simulink model "OCTModel_bandLin"  (R2020a)
settings: Solver=ode23s  StartTime=0.0  StopTime=simParams.duration.Value  FixedStep=0.1  MaxStep=0.1*sqrt(simParams.lengthScaleFactor.Value)  RelTol=1e-3  AbsTol=1e-3
undefined symbols (not defined in the file): ctrlFreeze, ctrlFreezeTime, linCtrl
libraries: simulink x3, pathFollowingControllerManta_cl x1, environment_cl x1, flightController_cl x1, gndStnController_cl x1, hiLvlController_cl x1, plant_cl x1, sensorProcessing_cl x1, sensors_cl x1
PreSaveFcn:
  | % Callback to reset the view so that the
  | % the next person to open isn't totally lost.
  | %hilite_system('OCTModel/plant');
  | %hilite_system('OCTModel/plant','none');
  | %set_param(gcs,'Zoomfactor','fit to view')
settings Model: PauseTimes=35  EnablePacing=on  PacingRate=56  ExtModeTrigDuration=100  Creator=mcobb  LastModifiedBy=andre
settings SolverCC: AlgebraicLoopSolver=LineSearch  SolverResetMethod=Robust
settings DataIOCC: SaveFinalState=on  SaveFormat=StructureWithTime  SaveOutput=off  DSMLogging=off  ReturnWorkspaceOutputs=off  StateSaveName=tmp_raccel_xout
settings OptimizationCC: EfficientMapNaN2IntZero=off
settings DebuggingCC: SignalRangeChecking=error  AlgebraicLoopMsg=none  ArtificialAlgebraicLoopMsg=none  ArithmeticOperatorsInVariantConditions=warning
settings HardwareCC: TargetBitPerPointer=64  TargetBitPerSizeT=64  TargetBitPerPtrDiffT=64  TargetLongLongMode=on  TargetIntDivRoundTo=Zero  TargetEndianess=LittleEndian  TargetWordSize=64  TargetHWDeviceType=MATLAB Host  ProdEqTarget=off
settings SFSimCC: CustomCodeUndefinedFunction=UseInterfaceOnly
settings CodeAppCC: MaxIdLength=128
settings GRTTargetCC: TargetLangStandard=C89/C90 (ANSI)  CombineOutputUpdateFcns=off  GRTInterface=on

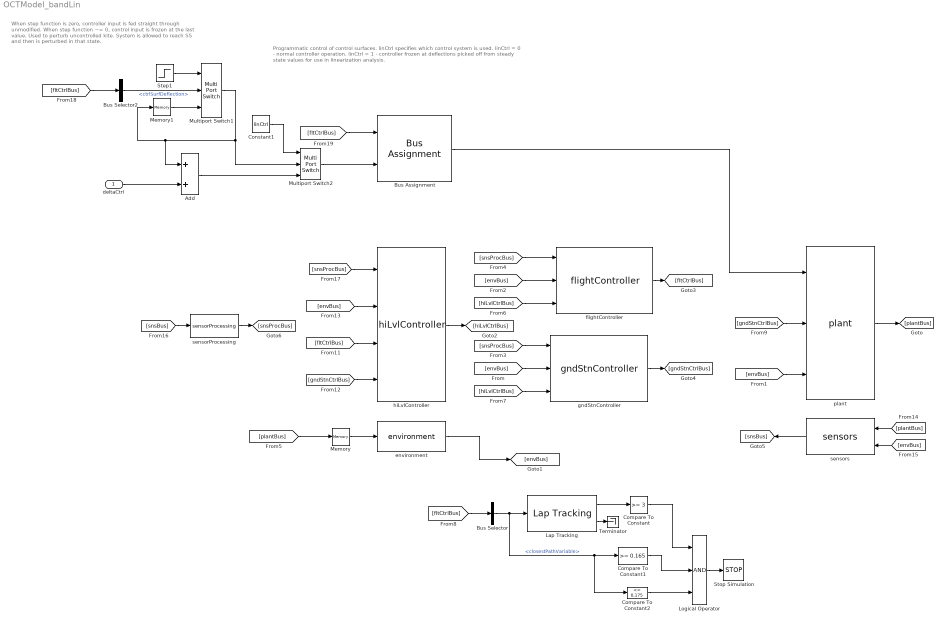
== system OCTModel_bandLin ==
  note: Programmatic control of control surfaces. linCtrl specifies which control  system is used.
      | linCtrl = 0 - normal controller operation. linCtrl = 1 - controller frozen at deflections picked off
      | from steady state values for use in linearization analysis.
  note: When step function is zero, controller input is fed straight through
      | unmodified. When step function ~= 0, control input is frozen at the
      | last value. Used to perturb uncontrolled kite. System is allowed to
      | reach SS and then is perturbed in that state.
  deltaCtrl : Inport  PortDimensions=4
  Add : Sum
  Bus Assignment : BusAssignment  AssignedSignals=ctrlSurfDeflection
  Bus Selector : BusSelector  OutputSignals=closestPathVariable
  Bus Selector2 : BusSelector  OutputSignals=ctrlSurfDeflection
  Compare To Constant : simulink/Logic and Bit Operations/Compare To Constant  relop=>=  const=3  OutDataTypeStr=boolean
  Compare To Constant1 : simulink/Logic and Bit Operations/Compare To Constant  relop=>=  const=0.165  OutDataTypeStr=boolean
  Compare To Constant2 : simulink/Logic and Bit Operations/Compare To Constant  relop=<=  const=0.175  OutDataTypeStr=boolean
  Constant1 : Constant  Value=linCtrl
  Lap Tracking : pathFollowingControllerManta_cl/pathFollowingControllerManta/Lap Tracking  SystemSampleTime=-1  Latency=0  AutoFrameSizeCalculation=off
  Logical Operator : Logic  Inputs=3  AllPortsSameDT=off  OutDataTypeStr=boolean
  Memory : Memory
  Memory1 : Memory  LinearizeMemory=on
  Multiport Switch1 : MultiPortSwitch  DataPortOrder=Zero-based contiguous  Inputs=2  zeroidx=on
  Multiport Switch2 : MultiPortSwitch  DataPortOrder=Zero-based contiguous  Inputs=2  zeroidx=on
  Step1 : Step  Time=ctrlFreezeTime  After=ctrlFreeze  SampleTime=0
  Stop Simulation : Stop
  Terminator : Terminator
  environment : environment_cl/environment  SystemSampleTime=-1  Latency=0  AutoFrameSizeCalculation=off
  flightController : flightController_cl/flightController  SystemSampleTime=-1  Latency=0  AutoFrameSizeCalculation=off
      link override slController/Roll//Yaw Controller/rollAzYawSide/Subsystem/1-D Lookup Table: BreakpointsForDimension1=[0 300 310 320 330]  Table=[0 0 10 0 0]
      link override slController/Roll//Yaw Controller/yawAz/Azimuth Control PID/Gain1: Gain=-1
      link override slController/Roll//Yaw Controller/yawAz/Setpoint PID Control/Gain1: Gain=-pi/180
      link override slController/Roll//Yaw Controller/yawAz/Step1: Time=600  After=-10
      link override slController/Roll//Yaw Controller/yawAz/Subsystem/1-D Lookup Table: BreakpointsForDimension1=[0 300 310 360 450]  Table=[0 0 10 0 0]
  gndStnController : gndStnController_cl/gndStnController  SystemSampleTime=-1  Latency=0  AutoFrameSizeCalculation=off
  hiLvlController : hiLvlController_cl/hiLvlController  SystemSampleTime=-1  Latency=0  AutoFrameSizeCalculation=off
  plant : plant_cl/plant  SystemSampleTime=-1  Latency=0  AutoFrameSizeCalculation=off
  sensorProcessing : sensorProcessing_cl/sensorProcessing  SystemSampleTime=-1  Latency=0  AutoFrameSizeCalculation=off
  sensors : sensors_cl/sensors  SystemSampleTime=-1  Latency=0  AutoFrameSizeCalculation=off
  wires:
  Memory/1 -> environment/1
  [envBus] -> gndStnController/2
  [snsProcBus] -> gndStnController/1
  [snsProcBus] -> flightController/1
  [snsProcBus] -> hiLvlController/1
  flightController/1 -> [fltCtrlBus]
  gndStnController/1 -> [gndStnCtrlBus]
  [envBus] -> hiLvlController/2
  [fltCtrlBus] -> hiLvlController/3
  [gndStnCtrlBus] -> hiLvlController/4
  [plantBus] -> Memory/1
  [hiLvlCtrlBus] -> flightController/3
  [hiLvlCtrlBus] -> gndStnController/3
  hiLvlController/1 -> [hiLvlCtrlBus]
  [envBus] -> flightController/2
  [plantBus] -> sensors/1
  [envBus] -> sensors/2
  sensors/1 -> [snsBus]
  [snsBus] -> sensorProcessing/1
  sensorProcessing/1 -> [snsProcBus]
  plant/1 -> [plantBus]
  Bus Assignment/1 -> plant/1
  [gndStnCtrlBus] -> plant/2
  [envBus] -> plant/3
  environment/1 -> [envBus]
  [fltCtrlBus] -> Bus Selector/1
  Bus Selector/1 -> Compare To Constant2/1, Compare To Constant1/1, Lap Tracking/1  "<closestPathVariable>"
  Lap Tracking/2 -> Terminator/1
  Lap Tracking/1 -> Compare To Constant/1
  Logical Operator/1 -> Stop Simulation/1
  Compare To Constant/1 -> Logical Operator/1
  Compare To Constant1/1 -> Logical Operator/2
  Compare To Constant2/1 -> Logical Operator/3
  Step1/1 -> Multiport Switch1/1
  Multiport Switch2/1 -> Bus Assignment/2
  [fltCtrlBus] -> Bus Assignment/1
  Bus Selector2/1 -> Multiport Switch1/2  "<ctrlSurfDeflection>"
  deltaCtrl/1 -> Add/2
  Multiport Switch1/1 -> Add/1, Memory1/1, Multiport Switch2/2
  Add/1 -> Multiport Switch2/3
  Memory1/1 -> Multiport Switch1/3
  [fltCtrlBus] -> Bus Selector2/1
  Constant1/1 -> Multiport Switch2/1
